simulink model "adcTestHarness"  (R2024a)
settings: configuration reference "standardSILConfiguraitonParams" (kept outside this file)
settings Model: Creator=aeroth  LastModifiedBy=UFC
settings ConfigSetRef: SourceName=standardSILConfiguraitonParams  SourceLocation=Base Workspace

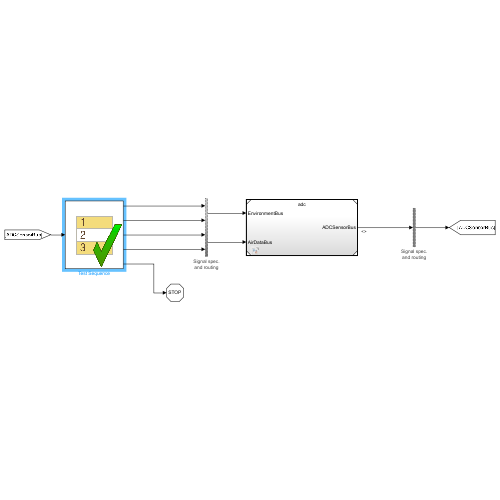
[thumbnail: Simulink's stored preview of the top-level diagram]
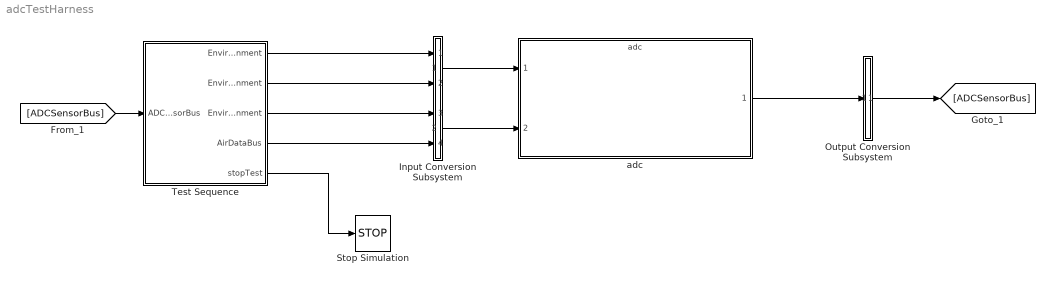
== system adcTestHarness ==
  Input Conversion Subsystem : Subsystem  Tag=__SLT_ICS__  Description=|
      | Signal spec.
      | and routing
      settings: AttributesFormatString=%<Description>
  Output Conversion Subsystem : Subsystem  Tag=__SLT_OCS__  Description=|
      | Signal spec.
      | and routing
      mask init:
      | ICDictionary = get_param(bdroot, 'DataDictionary');
      | if isempty(ICDictionary)
      |    ICScope = Simulink.data.BaseWorkspace;
      | else
      |    ICScope = Simulink.data.DataDictionary(ICDictionary);
      | end
      | 
      | IC1 = Simulink.Bus.createMATLABStruct('ADCSensorBus', [], [1 1], ICScope);
      settings: AttributesFormatString=%<Description>
  Stop Simulation : Stop
  Test Sequence : Test Sequence  TreatAsAtomicUnit=on
  adc : ModelReference  ModelNameDialog=adc  SimulationMode=Normal  ModelReferenceVersion=1.41
  wires:
  Test Sequence/1(EnvironmentBus_EarthEnvironment) -> Input Conversion Subsystem/1(Inport_1)
  Test Sequence/2(EnvironmentBus_AirEnvironment) -> Input Conversion Subsystem/2(Inport_2)
  Test Sequence/3(EnvironmentBus_TerrainEnvironment) -> Input Conversion Subsystem/3(Inport_3)
  Test Sequence/4(AirDataBus) -> Input Conversion Subsystem/4(Inport_4)
  [ADCSensorBus] -> Test Sequence/1(ADCSensorBus)
  Output Conversion Subsystem/1(Outport_1) -> [ADCSensorBus]
  Test Sequence/5(stopTest) -> Stop Simulation/1
  adc/1 -> Output Conversion Subsystem/1(Inport_1)
  Input Conversion Subsystem/1(Outport_1) -> adc/1
  Input Conversion Subsystem/2(Outport_2) -> adc/2

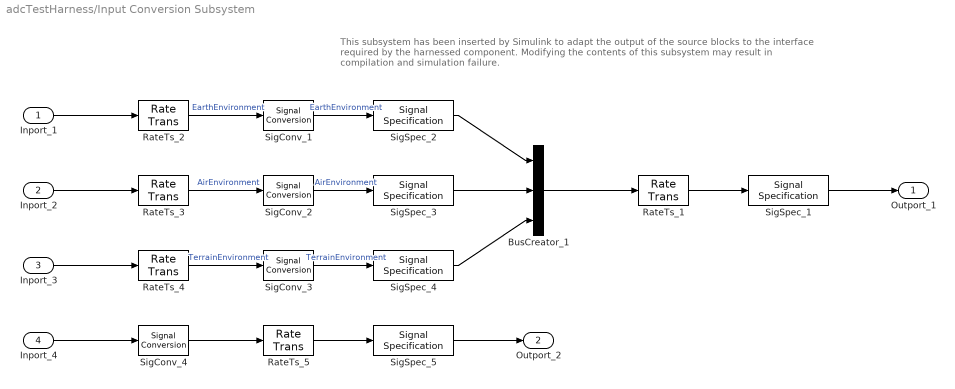
== system adcTestHarness/Input Conversion Subsystem ==
  note: This subsystem has been inserted by Simulink to adapt the output of the source blocks to the interface required by the harnessed component.
      |  Modifying the contents of this subsystem may result in compilation and simulation failure.
  Inport_1 : Inport
  Inport_2 : Inport  Port=2
  Inport_3 : Inport  Port=3
  Inport_4 : Inport  Port=4
  BusCreator_1 : BusCreator  Inputs=3  OutDataTypeStr=Bus: EnvironmentBus
  RateTs_{1..5} (5 alike) : RateTransition  OutPortSampleTime=0.004
  SigConv_1 : SignalConversion  ConversionOutput=Nonvirtual bus  OverrideOpt=off
  SigConv_2 : SignalConversion  ConversionOutput=Nonvirtual bus  OverrideOpt=off
  SigConv_3 : SignalConversion  ConversionOutput=Nonvirtual bus  OverrideOpt=off
  SigConv_4 : SignalConversion  ConversionOutput=Virtual bus  OverrideOpt=off
  SigSpec_1 : SignalSpecification  OutDataTypeStr=Bus: EnvironmentBus  SampleTime=0.004
  SigSpec_2 : SignalSpecification  OutDataTypeStr=Bus: EarthEnvironmentBus  Dimensions=[1]  SampleTime=0.004  BusOutputAsStruct=on
  SigSpec_3 : SignalSpecification  OutDataTypeStr=Bus: AirEnvironmentBus  Dimensions=[1]  SampleTime=0.004  BusOutputAsStruct=on
  SigSpec_4 : SignalSpecification  OutDataTypeStr=Bus: TerrainEnvironmentBus  Dimensions=[1]  SampleTime=0.004  BusOutputAsStruct=on
  SigSpec_5 : SignalSpecification  OutDataTypeStr=Bus: AirData  SampleTime=0.004
  Outport_1 : Outport
  Outport_2 : Outport  Port=2
  wires:
  SigSpec_1/1 -> Outport_1/1
  RateTs_1/1 -> SigSpec_1/1
  BusCreator_1/1 -> RateTs_1/1
  SigSpec_2/1 -> BusCreator_1/1
  SigConv_1/1 -> SigSpec_2/1  "EarthEnvironment"
  RateTs_2/1 -> SigConv_1/1  "EarthEnvironment"
  Inport_1/1 -> RateTs_2/1
  SigSpec_3/1 -> BusCreator_1/2
  SigConv_2/1 -> SigSpec_3/1  "AirEnvironment"
  RateTs_3/1 -> SigConv_2/1  "AirEnvironment"
  Inport_2/1 -> RateTs_3/1
  SigSpec_4/1 -> BusCreator_1/3
  SigConv_3/1 -> SigSpec_4/1  "TerrainEnvironment"
  RateTs_4/1 -> SigConv_3/1  "TerrainEnvironment"
  Inport_3/1 -> RateTs_4/1
  SigSpec_5/1 -> Outport_2/1
  RateTs_5/1 -> SigSpec_5/1
  SigConv_4/1 -> RateTs_5/1
  Inport_4/1 -> SigConv_4/1

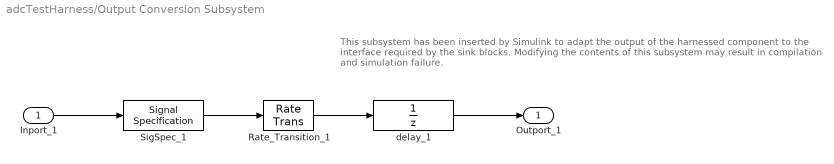
== system adcTestHarness/Output Conversion Subsystem ==
  note: This subsystem has been inserted by Simulink to adapt the output of the harnessed component to the interface required by the sink blocks.
      |  Modifying the contents of this subsystem may result in compilation and simulation failure.
  Inport_1 : Inport
  Rate_Transition_1 : RateTransition  OutPortSampleTimeOpt=Inherit
  SigSpec_1 : SignalSpecification  OutDataTypeStr=Bus: ADCSensorBus  Dimensions=[1]  SampleTime=0.004
  delay_1 : UnitDelay  InitialCondition=IC1  SampleTime=-1
  Outport_1 : Outport
  wires:
  Inport_1/1 -> SigSpec_1/1
  SigSpec_1/1 -> Rate_Transition_1/1
  Rate_Transition_1/1 -> delay_1/1
  delay_1/1 -> Outport_1/1

== stateflow chart adcTestHarness/Test Sequence ==
  state Scenario_1
    state Initialize
      stopTest = false;
      %% Initialize data outputs.
      EnvironmentBus_EarthEnvironment.gravityScalar_mps2 = 9.81;
      EnvironmentBus_AirEnvironment.airTemperature_K = 288.15; %standard, 15deg C
      EnvironmentBus_AirEnvironment.airPressure_Pa = 101325; %standard
      EnvironmentBus_AirEnvironment.airDensity_kgpm3 = 1.225; %kgpm3 at 15 deg C
      EnvironmentBus_AirEnvironment.windSpeedInNED_mps = zeros(3,1);
      EnvironmentBus_AirEnvironment.speedOfSound_mps = 340.3;
      EnvironmentBus_TerrainEnvironment.terrainHeightInNED_m = 0;
      AirDataBus.airspeedInBody_mps = zeros(3,1);
      AirDataBus.alpha_rad = 0;
      AirDataBus.beta_rad = 0;
    state checkSensors
      verify(isClose(ADCSensorBus.BaroSensorBus.altitude_m, 0, 'atol', 20)) %check baro altitude is ~0 MSL
      verify(isClose(ADCSensorBus.BaroSensorBus.pressure_pa, 101325, 'atol', 100))
      verify(isClose(ADCSensorBus.BaroSensorBus.temperature_degC, 15, 'atol', 2))
      verify(isClose(ADCSensorBus.DiffPressureSensorBus.differential_pressure_pa, 0, 'atol', 100))
      verify(isClose(ADCSensorBus.DiffPressureSensorBus.temperature_degC, 15, 'atol', 2))
    state check10kft
      EnvironmentBus_AirEnvironment.airTemperature_K = 268;  %standard @ 20 kft
      EnvironmentBus_AirEnvironment.airPressure_Pa = 69681.66; %standard
      EnvironmentBus_AirEnvironment.airDensity_kgpm3 = 0.4135; %kgpm3
      EnvironmentBus_AirEnvironment.windSpeedInNED_mps = zeros(3,1);
      EnvironmentBus_AirEnvironment.speedOfSound_mps = 328.4;
    state checkSensors10kft
      verify(isClose(ADCSensorBus.BaroSensorBus.altitude_m, 3048, 'atol', 20)) %check baro altitude is ~0 MSL
      verify(isClose(ADCSensorBus.BaroSensorBus.pressure_pa,  69681.66, 'atol', 100))
      verify(isClose(ADCSensorBus.BaroSensorBus.temperature_degC, -4.8, 'atol', 2))
      verify(isClose(ADCSensorBus.DiffPressureSensorBus.differential_pressure_pa, 0, 'atol', 100))
      verify(isClose(ADCSensorBus.DiffPressureSensorBus.temperature_degC, -4.8, 'atol', 2))
    state check20kft
      EnvironmentBus_AirEnvironment.airTemperature_K = 248; %standard @ 20 kft
      EnvironmentBus_AirEnvironment.airPressure_Pa = 46563.26; %standard
      EnvironmentBus_AirEnvironment.airDensity_kgpm3 = 0.3639; %kgpm3
      EnvironmentBus_AirEnvironment.windSpeedInNED_mps = zeros(3,1);
      EnvironmentBus_AirEnvironment.speedOfSound_mps = 316;
    state checkSensors20kft
      verify(isClose(ADCSensorBus.BaroSensorBus.altitude_m, 6096, 'atol', 20)) %check baro altitude is ~0 MSL
      verify(isClose(ADCSensorBus.BaroSensorBus.pressure_pa,  46563.26, 'atol', 100))
      verify(isClose(ADCSensorBus.BaroSensorBus.temperature_degC, -24.624, 'atol', 2))
      verify(isClose(ADCSensorBus.DiffPressureSensorBus.differential_pressure_pa, 0, 'atol', 100))
      verify(isClose(ADCSensorBus.DiffPressureSensorBus.temperature_degC, -24.624, 'atol', 2))
    state addAirspeed
      AirDataBus.airspeedInBody_mps = [100 0 0]';
    state checkDiffPress
      verify(ADCSensorBus.DiffPressureSensorBus.differential_pressure_pa > 0) %TODO: check sign on diff press and check with alpha, beta once model is updated to use these
    state EndTest
      stopTest = true;
    (default) -> Initialize
    Initialize -> checkSensors : [
        | true
        | ]
    checkSensors -> check10kft : [
        | true
        | ]
    check10kft -> checkSensors10kft : [
        | true
        | ]
    checkSensors10kft -> check20kft : [
        | true
        | ]
    check20kft -> checkSensors20kft : [
        | true
        | ]
    checkSensors20kft -> addAirspeed : [
        | true
        | ]
    addAirspeed -> checkDiffPress : [
        | true
        | ]
    checkDiffPress -> EndTest : [
        | true
        | ]
  (default) -> Scenario_1 : {assert(Active_Scenario_Index == 1,'The value of Scenario Parameter ''Active_Scenario_Index'' is not valid. Use the index of the scenario to specify it.')}
  data: ADCSensorBus input Bus: ADCSensorBus size=[1]; EnvironmentBus_EarthEnvironment output Bus: EarthEnvironmentBus size=[1]; EnvironmentBus_AirEnvironment output Bus: AirEnvironmentBus size=[1]; EnvironmentBus_TerrainEnvironment output Bus: TerrainEnvironmentBus size=[1]; AirDataBus output Bus: AirData size=[1]; Active_Scenario_Index parameter =1; stopTest output
